simulink model "zad1_sim"  (R2025a)
settings: Solver=VariableStepAuto  StartTime=0.0  StopTime=10.0  RelTol=1e-3
values from neighbouring files (symbols this model uses):
  A = [0            0        1            0 ... (first row only)    [zad1.m]
  B = [c1/m1 ... (first row only)    [zad1.m]
  C = [1 0 0 0]    [zad1.m]
  c1 = 100    [zad1.m]
  c2 = 2000    [zad1.m]
  D = 0    [zad1.m]
  k1 = 370000    [zad1.m]
  k2 = 35000    [zad1.m]
  m1 = 90    [zad1.m]
  m2 = 600    [zad1.m]
settings Model: Creator=Dejmian  LastModifiedBy=Dejmian

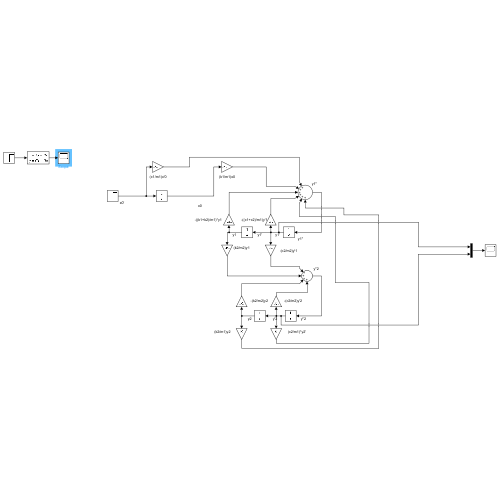
[thumbnail: Simulink's stored preview of the top-level diagram]
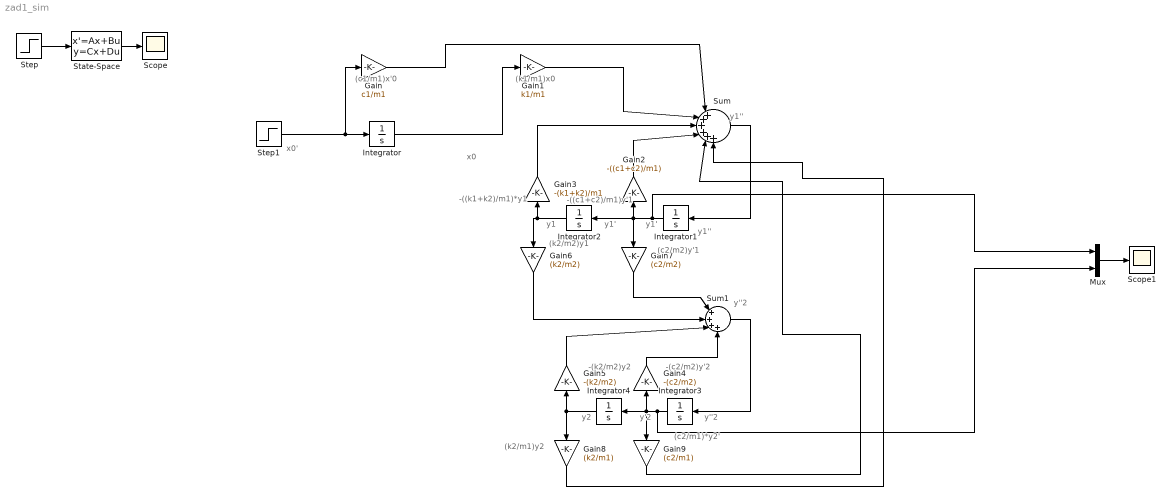
== system zad1_sim ==
  note: (c2/m1)*y2'
  note: (k2/m1)y2
  note: (c2/m2)y'1
  note: (k2/m2)y1
  note: -(k2/m2)y2
  note: -(c2/m2)y'2
  note: y2
  note: y'2
  note: y''2
  note: y''2
  note: -((c1+c2)/m1)y'1
  note: -((k1+k2)/m1)*y1
  note: y1'
  note: y1
  note: y1'
  note: y1''
  note: y1''
  note: (c1/m1)x'0
  note: (k1/m1)x0
  note: x0
  note: x0'
  Gain : Gain  Gain=c1/m1
  Gain1 : Gain  Gain=k1/m1
  Gain2 : Gain  Gain=-((c1+c2)/m1)
  Gain3 : Gain  Gain=-(k1+k2)/m1
  Gain4 : Gain  Gain=-(c2/m2)
  Gain5 : Gain  Gain=-(k2/m2)
  Gain6 : Gain  Gain=(k2/m2)
  Gain7 : Gain  Gain=(c2/m2)
  Gain8 : Gain  Gain=(k2/m1)
  Gain9 : Gain  Gain=(c2/m1)
  Integrator{,1..4} (5 alike) : Integrator
  Mux : Mux  Inputs=2
  Scope : Scope
      settings: ActiveDisplayYMinimum=-2.041582880816077  ActiveDisplayYMaximum=3.9609612128569687
  Scope1 : Scope
      settings: ActiveDisplayYMinimum=-1  ActiveDisplayYMaximum=1
  State-Space : StateSpace  A=A  B=B  C=C  D=D  InitialCondition=0
  Step : Step  SampleTime=0
  Step1 : Step  SampleTime=0
  Sum : Sum  Inputs=|++++++
  Sum1 : Sum  Inputs=|++++
  wires:
  Step/1 -> State-Space/1
  Step1/1 -> Gain/1, Integrator/1
  Integrator/1 -> Gain1/1
  Gain1/1 -> Sum/2
  Gain/1 -> Sum/1
  Sum/1 -> Integrator1/1
  Integrator1/1 -> Mux/1, Gain7/1, Gain2/1, Integrator2/1
  Integrator2/1 -> Gain6/1, Gain3/1
  Gain3/1 -> Sum/3
  Gain2/1 -> Sum/4
  Integrator3/1 -> Mux/2, Gain9/1, Gain4/1, Integrator4/1
  Sum1/1 -> Integrator3/1
  Gain4/1 -> Sum1/4
  Integrator4/1 -> Gain8/1, Gain5/1
  Gain5/1 -> Sum1/3
  Gain6/1 -> Sum1/2
  Gain7/1 -> Sum1/1
  Gain8/1 -> Sum/6
  Gain9/1 -> Sum/5
  Mux/1 -> Scope1/1
  State-Space/1 -> Scope/1
